simulink model "UAVNLCL_TRACK_GS_5D"  (R2023a)
settings: Solver=ode45  StartTime=0.0  StopTime=30  MaxStep=0.4  RelTol=1e-3  EnableMultiTasking=on
values from neighbouring files (symbols this model uses):
  Ct = [0, 0, 0, 0, 1]    [PI_6_Tracker_GS.m]    (also in PI_6_Tracker_bigGuy.m)
  IP = 0.1568    [PI_3_GenerateDataset.m]
  K2 = Kt(:,6)    [PI_6_Tracker_GS.m]    (also in PI_6_Tracker_bigGuy.m)
  Ks_range = zeros(2,5*size(Vs_range,2))    [PI_6_Tracker_bigGuy.m]
  slopes = [0, rawslopes(2)]    [PI_6_Tracker_GS.m]    (also in PI_6_Tracker_bigGuy.m)
  TABLEDATA = [1.10335162023 0.00823171458117 -11.0555848055 -0.375153780134 6.18853169798 -34.1001082535 0.0324757076966 -9.89122049893 0.729242255451 -0.683674300952 1.08721495624 0.00509823507416 ... (12710 elements, 2x5x41x31)]    [TableData_002.mat]    (also in TableData_004.mat = [0.174322085341 -0.0514346863342 -0.753716023023 2.529946466; TableData_006.mat = [0.237084016899 -0.0298197541441 -1.42090322153 1.5613882815; TableData_007GS.mat = [0.237084016899 -0.0298197541441 -1.42090322153 1.5613882815; TableData_009.mat = [0.235717817503 -0.0298554739715 -1.40805314109 1.5648466906)
  Vs_range = [10; 45]    [PI_6_Tracker_bigGuy.m]
  W = 2.5    [Calculos00_OriginalIgnacio.m]    (also in Calculos02_Vnoladetrim.m; Calculos03_TablaTrimados.m; GenerateDataset_v0.m; PI_0_OnlyOneController_V20.m)
  x0t = zeros(5,1)    [PI_6_Tracker_GS.m]    (also in PI_6_Tracker_bigGuy.m)
  XCG = 0.33    [Calculos00_OriginalIgnacio.m]    (also in Calculos02_Vnoladetrim.m; Calculos03_TablaTrimados.m; GenerateDataset_v0.m; PI_0_OnlyOneController_V20.m)
undefined symbols (not defined in the file or in its folder): Utrim, Xtrim
libraries: simulink x4, simulink_extras x1
settings Model: SimulationMode=accelerator  Creator=Ignacio  LastModifiedBy=ignac
settings SolverCC: AlgebraicLoopSolver=TrustRegion
settings DataIOCC: ExternalInput=[0 0.369809473744665 -0.0760167506859634 0.299999999999976]  InitialState=[]  LimitDataPoints=on  SaveFormat=Array  SignalLoggingSaveFormat=ModelDataLogs  ReturnWorkspaceOutputs=off
settings OptimizationCC: DefaultParameterBehavior=Inlined  BufferReuse=off  ExpressionDepthLimit=2147483647  LifeSpan=inf
settings DebuggingCC: UnderspecifiedInitializationDetection=Classic  MergeDetectMultiDrivingBlocksExec=none  FcnCallInpInsideContextMsg=warning  UnconnectedInputMsg=warning  UnconnectedOutputMsg=warning  UnconnectedLineMsg=warning  StateNameClashWarn=warning  InitInArrayFormatMsg=none  SFUnexpectedBacktrackingDiag=warning  SFNoUnconditionalDefaultTransitionDiag=warning  SFExecutionAtInitializationDiag=none  ArithmeticOperatorsInVariantConditions=warning
settings HardwareCC: ProdBitPerPointer=32  ProdBitPerSizeT=32  ProdBitPerPtrDiffT=32  ProdLargestAtomicFloat=None  ProdIntDivRoundTo=Undefined  ProdEndianess=Unspecified  ProdWordSize=32  ProdHWDeviceType=32-bit Generic
settings ModelReferenceCC: EnableRefExpFcnMdlSchedulingChecks=on  PropagateSignalLabelsOutOfModel=off
settings SFSimCC: SimUseLocalCustomCode=off  CustomCodeUndefinedFunction=UseInterfaceOnly
settings RTWCC: RTWUseLocalCustomCode=off
settings CodeAppCC: StateflowObjectComments=on
settings GRTTargetCC: TargetLangStandard=C89/C90 (ANSI)
settings ConfigComp: CovMetricSettings=dw  CovSaveCumulativeToWorkspaceVar=on  CovSaveSingleToWorkspaceVar=on  CovExternalEMLEnable=off

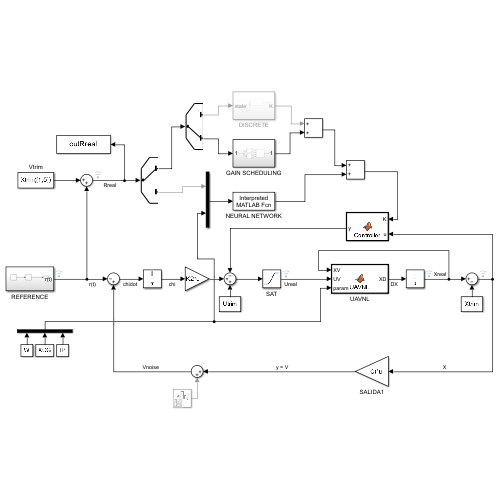
[thumbnail: Simulink's stored preview of the top-level diagram]
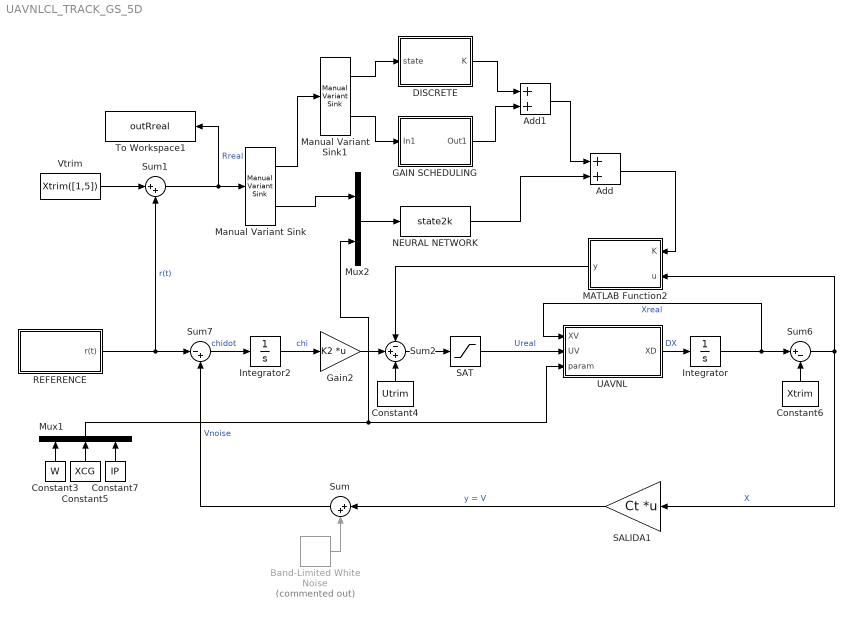
== system UAVNLCL_TRACK_GS_5D ==
  Add : Sum
  Add1 : Sum
  Band-Limited White Noise : simulink/Sources/Band-Limited White Noise  Commented=on  Cov=[0.1]*0  Ts=0.1  seed=[23341]
  Constant3 : Constant  Value=W
  Constant4 : Constant  Value=Utrim
  Constant5 : Constant  Value=XCG
  Constant6 : Constant  Value=Xtrim
  Constant7 : Constant  Value=IP
  DISCRETE : Subsystem
  GAIN SCHEDULING : Subsystem
  Gain2 : Gain  Gain=K2  Multiplication=Matrix(K*u)
  Integrator : Integrator  InitialCondition=Xtrim+x0t  AbsoluteTolerance=-1
  Integrator2 : Integrator
  MATLAB Function2 : MATLAB Function  TreatAsAtomicUnit=on
  Manual Variant Sink : simulink/Signal Routing/Manual Variant Sink  NumChoices=2  LabelModeActiveChoice=V_1
  Manual Variant Sink1 : simulink/Signal Routing/Manual Variant Sink  NumChoices=2  LabelModeActiveChoice=V_2
  Mux1 : Mux  Inputs=3
  Mux2 : Mux  Inputs=2
  NEURAL NETWORK : MATLABFcn  MATLABFcn=state2k  OutputDimensions=[2,5]  Output1D=off
  REFERENCE : Subsystem
  SALIDA1 : Gain  Gain=Ct  Multiplication=Matrix(K*u)
  SAT : Saturate  UpperLimit=[1; 0.5]  LowerLimit=[0; -0.5]
  Sum : Sum  Inputs=|++
  Sum1 : Sum  Inputs=|++
  Sum2 : Sum  Inputs=-++
  Sum6 : Sum  Inputs=|+-
  Sum7 : Sum  Inputs=|-+
  To Workspace1 : ToWorkspace  VariableName=outRreal  SaveFormat=Timeseries  SampleTime=-1
      settings: Save2DSignal=2-D array (concatenate along first dimension)
  UAVNL : MATLAB Function  TreatAsAtomicUnit=on
  Vtrim : Constant  Value=Xtrim([1,5])
  wires:
  UAVNL/1(XD) -> Integrator/1  "DX"
  Integrator/1 -> Sum6/1, UAVNL/1(XV)  "Xreal"
  Band-Limited White Noise/1 -> Sum/2
  Constant6/1 -> Sum6/2
  Sum6/1 -> MATLAB Function2/2(u), SALIDA1/1  "X"
  SAT/1 -> UAVNL/2(UV)  "Ureal"
  SALIDA1/1 -> Sum/1  "y = V"
  Sum7/1 -> Integrator2/1  "chidot"
  Integrator2/1 -> Gain2/1  "chi"
  Sum/1 -> Sum7/2  "Vnoise"
  Gain2/1 -> Sum2/2
  Constant4/1 -> Sum2/3
  MATLAB Function2/1(y) -> Sum2/1
  Sum2/1 -> SAT/1
  Vtrim/1 -> Sum1/1
  Add/1 -> MATLAB Function2/1(K)
  NEURAL NETWORK/1 -> Add/2
  Sum1/1 -> To Workspace1/1, Manual Variant Sink/1  "Rreal"
  Manual Variant Sink/1 -> Manual Variant Sink1/1
  Manual Variant Sink1/1 -> DISCRETE/1(state)
  Manual Variant Sink1/2 -> GAIN SCHEDULING/1(In1)
  DISCRETE/1(K) -> Add1/1
  GAIN SCHEDULING/1(Out1) -> Add1/2
  Add1/1 -> Add/1
  REFERENCE/1(r(t)) -> Sum7/1, Sum1/2  "r(t)"
  Constant5/1 -> Mux1/2
  Constant3/1 -> Mux1/1
  Constant7/1 -> Mux1/3
  Mux1/1 -> Mux2/2, UAVNL/3(param)
  Manual Variant Sink/2 -> Mux2/1
  Mux2/1 -> NEURAL NETWORK/1

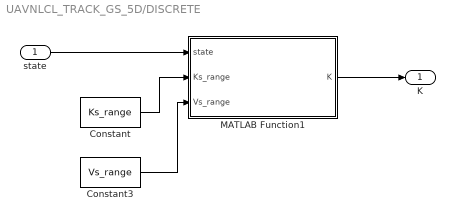
== system UAVNLCL_TRACK_GS_5D/DISCRETE ==
  state : Inport
  Constant : Constant  Value=Ks_range
  Constant3 : Constant  Value=Vs_range
  MATLAB Function1 : MATLAB Function  TreatAsAtomicUnit=on
  K : Outport
  wires:
  Constant/1 -> MATLAB Function1/2(Ks_range)
  Constant3/1 -> MATLAB Function1/3(Vs_range)
  state/1 -> MATLAB Function1/1(state)
  MATLAB Function1/1(K) -> K/1

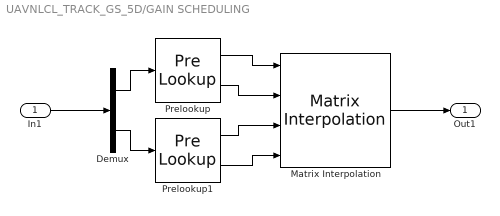
== system UAVNLCL_TRACK_GS_5D/GAIN SCHEDULING ==
  In1 : Inport
  Demux : Demux  Outputs=2
  Matrix Interpolation : simulink_extras/Additional Lookup Tables/Matrix Interpolation  InterpMethod=Linear  ExtrapMethod=Clip  InterpolateDimension=2  TableData=TABLEDATA  SimulateUsing=Code generation
  Prelookup : PreLookup  BreakpointsData=vV  ExtrapMethod=Linear
  Prelookup1 : PreLookup  BreakpointsData=vH  ExtrapMethod=Linear
  Out1 : Outport
  wires:
  Demux/1 -> Prelookup/1
  In1/1 -> Demux/1
  Matrix Interpolation/1 -> Out1/1
  Demux/2 -> Prelookup1/1
  Prelookup/2 -> Matrix Interpolation/2
  Prelookup/1 -> Matrix Interpolation/1
  Prelookup1/1 -> Matrix Interpolation/3
  Prelookup1/2 -> Matrix Interpolation/4

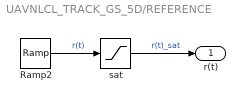
== system UAVNLCL_TRACK_GS_5D/REFERENCE ==
  Ramp2 : simulink/Sources/Ramp  slope=slopes  start=0  InitialOutput=0*slopes
  sat : Saturate  UpperLimit=slopes*20  LowerLimit=0*slopes
  r(t) : Outport
  wires:
  Ramp2/1 -> sat/1  "r(t)"
  sat/1 -> r(t)/1  "r(t)_sat"

== matlab function UAVNLCL_TRACK_GS_5D/DISCRETE/MATLAB Function1 ==
  data: state input; K output; Ks_range input; Vs_range input
function K = state2k_discrete(state, Ks_range, Vs_range)
    % state = [V, H] instantánea
    % Ks_range = [K1, K2, K3, ...], con sus dimensiones (2,5,[])
    % Vs_range = [[V_start1;V_end1], [V_start2;V_end2],...]
    % El rango de V en el que va el controlador K3 es entre Vs_range(1,3) y
    % Vs_range(2,3).
    % K2 se usa entre [V_start2, V_end2).
    % Ejemplo: Para tener un controlador K1 entre 10 y 15 m/s, otro K2 entre
    % los 15 y los 20, otro K3 entre 20 y 25 y K4 entre 25 y 30 m/s, argumentos:
    % Ks_range = [K1, K2, K3, K4]
    % Vs_range = [[10; 15], [15;20], [20;25], [25;30]];
    
    V = state(1);
    % H = state(2);

    K = zeros(2,5);

    Ks = reshape(Ks_range,2,5,[]);
    found = 0;

    for i = 1:size(Vs_range,2)
        range = Vs_range(:,i);
        if V >= range(1) && V < range(2)
            K = Ks(:,:,i);
            found = 1;
            disp(i)
        end
    end

    if ~found
        K = zeros(2,5);
        disp('ERROR: state2k_discrete: Range not satisfied.')
    end
end

== matlab function UAVNLCL_TRACK_GS_5D/MATLAB Function2 ==
  data: K input; u input; y output
function y = Controller(K,u)
    y = K*u;

== matlab function UAVNLCL_TRACK_GS_5D/UAVNL ==
  data: XV input; XD output; UV input; param input
function XD = UAVNL(XV,UV,param)

XD=zeros(5,1); % Inicializamos el vector de las derivadas con ceros

% DATOS DE LA AERONAVE

S = 0.4121;               % superficie alar (m^2)
C=0.2192;                  % cuerda media aerodinámica (m)
MASA=2.5;                  % Masa (Kg)
XCGR=0.33;                % posición de referencia del CG
IP=0.156794;                   % Momento de inercia (Kg*m^2)
d=1.225;                      % densidad (Kg/m^3)
G=9.8;                    % gravedad m/s^2
XCG=.33;                  % CG no coincide con el de referencia

% derivadas de estabilidad y control adimensionales

CLalpha0=0.405;    
CLalpha=5.379292;
CLq=11.133615;
CD0=0.0277;
CDalpha=0.14897;
CDalpha2=0.9848;
Cm0=0.0418;     
Cmalpha=-6.0; %1.812981 Más inestable en cabeceo
Cmalphadot=-7.0;
Cmde=-1.552;
Cmq=-18.422237;

% variables de estado


VT=XV(1);	% Velocidad 
ALPHA=XV(2);	% Angulo de ataque
THETA=XV(3);% Angulo de asiento
Q=XV(4);	% Velocidad angular de cabeceo
H=XV(5);

% variables de control

Dt=UV(1);	% Acelerador
De=UV(2);	% Deflexión del timón de profundidad

% parameters

MASA=param(1);
XCG=param(2);

% Density at altitude H
d=density(H);

% Algunos calculos previos

U=VT*cos(ALPHA);	% Componentes de la velocidad en ejes cuerpo
W=VT*sin(ALPHA);	

PDS=0.5*d*(VT^2)*S;	% Presión dinámica*Superficie alar

% Parametros Grupo Motopropulsor

Dh=0.254;   % Diametro de la helice (m)

REVmax=222; % Revoluciones maximas del motor (rev/s)

CT0=0.13805; % Coeficientes de traccion
CTj=-0.2049;
REV=REVmax*Dt; % Motor instantaneo
J=VT/(REV*Dh);  %Coef de velocidad
C_T=CT0+CTj*J;          %Coef de traccion
T=C_T*d*REV^2*Dh^4;     %Traccion

% coeficientes adimensionales de fuerzas y momentos (ejes viento)

CLT=CLalpha0+CLalpha*ALPHA+CLq*Q*C*0.5/VT;         
CDT=CD0+CDalpha*ALPHA+CDalpha2*ALPHA^2;  
CZ=-CDT*sin(ALPHA)-CLT*cos(ALPHA); % Cz en ejes cuerpo para añadir despues el efecto del centro de gravedad
CmT=Cm0+(Cmalpha*ALPHA)+(Cmde*De)+(CZ*(XCG-XCGR))+(C*0.5*Cmq*Q/VT); % Falta la componente alphadot,la añadiremos despues

% Fuerzas aerodinámicas

L=CLT*PDS;
D=CDT*PDS;

% Sistema de ecuaciones diferenciales de la dinámica del vuelo


UDOT=-Q*W+(T-MASA*G*sin(THETA)-D*cos(ALPHA)+L*sin(ALPHA))/MASA;
WDOT=Q*U+(MASA*G*cos(THETA)-D*sin(ALPHA)-L*cos(ALPHA))/MASA;
ALPHADOT=((U*WDOT-W*UDOT)/VT^2);
CmT=CmT+Cmalphadot*C/(2*VT)*ALPHADOT; % Completamos Cm
QDOT=CmT*PDS*C/IP;

VTDOT=(U*UDOT+W*WDOT)/VT;

% Construimos el vector con las derivadas de las variables de estado


XD(1)=VTDOT;
XD(2)=ALPHADOT;
XD(3)=Q;
XD(4)=QDOT;
XD(5)=VT*sin(THETA-ALPHA);
